simulink model "W3Q1"  (R2019b)
settings: Solver=VariableStepAuto  StartTime=0.0  StopTime=10.0  RelTol=1e-3
settings Model: Creator=Vinayak  LastModifiedBy=Vinayak

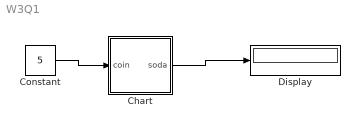
== system W3Q1 ==
  Chart : Stateflow chart  BlockKeywords=__PRM__SERIALIZED__DATA__:Stateflow Chart,Stateflow Diagram  TreatAsAtomicUnit=on
  Constant : Constant  Value=5
  Display : Display
  wires:
  Constant/1 -> Chart/1(coin)
  Chart/1(soda) -> Display/1

== stateflow chart W3Q1/Chart ==
  state received_0
  state received_5
  state received_10
  (default) -> received_0
  received_0 -> received_5 [order 1] : [coin==5]{soda=0}
  received_5 -> received_0 [order 1] : [coin==10]{soda=1}
  received_10 -> received_0 [order 1] : [coin==5]{soda=1}
  received_0 -> received_10 [order 2] : [coin==10]{soda=0}
  received_5 -> received_10 [order 2] : [coin==5]{soda=0}
  received_10 -> received_5 [order 2] : [coin==10]{soda=1}
  data: coin input; soda output
